simulink library "r2daq_blocks"  (R2012b)
settings: Solver=ode45  StartTime=0.0  StopTime=10.0  RelTol=1e-3
undefined symbols (not defined in the file or in its folder): biquad_iir, feedback_iir, filters, libddc, sfp, synth, xlfir_8x16
libraries: xbsIndex_r4 x4087, casper_library_misc x21, dspsigops x16, casper_library_delays x10, xps_library x1
(part 1 of 23)
settings Model: Creator=ayoung  LastModifiedBy=brent

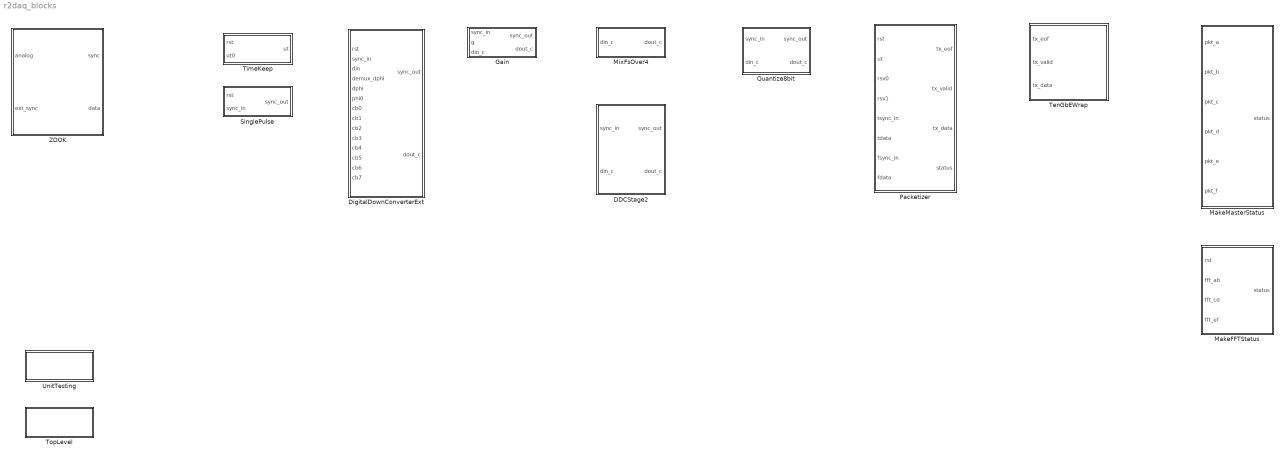
== system r2daq_blocks ==
  DDCStage2 : Subsystem
  DigitalDownConverterExt : Subsystem
  Gain : Subsystem
  MakeFFTStatus : Subsystem
  MakeMasterStatus : Subsystem
  MixFsOver4 : Subsystem
  Packetizer : Subsystem  mask(Packetizer){N_fft=8192, frames_per_batch=390625, IF_ID=1, Digital_ID=3, pd_in=3, pd_tvf=32}
      mask prompts: N_fft "FFT-size"; frames_per_batch "Frames in batch"; IF_ID "IF ID (6-bit)"; Digital_ID "Digital ID (6-bit)"; pd_in "Pipeline delay registers"; pd_tvf "Time packet delay relative to frequency packet"
      mask help:
      | Packetizes simultaneous time- and frequency-domain data for transmission using a 10GbE core.
      |
      | An asynchronous reset port is available as rst.
      |
      | Complex-valued frequency-domain data is supplied as UFix_16_0 to fdata. A single pulse on fsync_in indicates that the first sample of valid data will appear at fdata on the next clock cycle. Only one such pulse should be given per reset. The same applies to tdata and tsync_in.
      |
      | Current unix-time can be supplied as a UFix_32_0 to port ut.
      |
      | 64bit-wide header data can be supplied to each rsv0 and rsv1. Note that b63 (msb) of rsv1 is over-written internally.
      |
      | Signals to drive a 10GbE core are directly available in tx_eof, tx_valid, and tx_data.
      |
      | Empty and full signals of internal FIFO's used to buffer time- and frequency-domain data are available in ffifo_empty, ffifo_full, tfifo_empty and tfifo_full.
      mask init:
      | pd_inst = {...
      |     [gcb '/pd_ud0'],...
      |     [gcb '/pd_ud1']};
      | pd_in = get_param(gcb,'pd_in');
      | for ii=1:numel(pd_inst)
      |     set_param(pd_inst{ii},'latency',pd_in);
      | end
      | pd_inst = [gcb '/pd_dtf'];
      | %pd_tvf = get_param(gcb,'pd_tvf');
      | %set_param(pd_inst,'latency',pd_tvf);
      | pd_tvf_delay = 4;
      | set_param([gcb '/data_per_frame'],'const',num2str(N_fft-1));
      | set_param([gcb '/fpb_const'],'const',num2str(frames_per_batch));
      | set_param([gcb '/pd_dtf_pre'],'latency',num2str(pd_tvf_delay));
      | set_param([gcb '/delay_neg_edge'],'latency',num2str(pd_tvf-2*pd_tvf_delay));
      | set_param([gcb '/pd_dtf_post'],'latency',num2str(pd_tvf_delay));
  Quantize8bit : Subsystem  mask(Quantize8bit){pd_io=0}
      mask prompts: pd_io "Pipeline delay"
      mask help:
      | Quantize complex-valued input to Fix_8_7 by slicing top 8bits from each component.
      |
      | Pipeline delay is configurable.
      mask init:
      | pd_inst = {...
      |     [gcb '/pd_sync'],...
      |     [gcb '/pd_data']};
      | pd_io = get_param(gcb,'pd_io');
      | for ii=1:numel(pd_inst)
      |     set_param(pd_inst{ii},'latency',pd_io);
      | end
  SinglePulse : Subsystem
  TenGbEWrap : Subsystem  mask(TenGbEWrap){pd_in=3, pd_out=3}
      mask prompts: pd_in "Registers in pipeline delay"; pd_out "Registers out pipeline delay"
      mask help:
      | Wrap 10GbE core and supplies control and status registers internally.
      |
      | Pipeline delay to and from registers are configurable.
      mask init:
      | pd_inst = {...
      |     [gcb '/pd_ctrl'],...
      |     [gcb '/pd_port'],...
      |     [gcb '/pd_ip']};
      | pd_in = get_param(gcb,'pd_in');
      | for ii=1:numel(pd_inst)
      |     set_param(pd_inst{ii},'latency',pd_in);
      | end
      | pd_inst = {...
      |     [gcb '/pd_status']};
      | pd_out = get_param(gcb,'pd_out');
      | for ii=1:numel(pd_inst)
      |     set_param(pd_inst{ii},'latency',pd_out);
      | end
  TimeKeep : Subsystem
  TopLevel : Subsystem
      settings: OpenFcn=top_level
  UnitTesting : Subsystem
      settings: OpenFcn=unit_testing
  ZDOK : Subsystem  mask{zdok_slot=ZDOK 1, freq_nyq=1600}
      mask prompts: zdok_slot "ZDOK slot"; freq_nyq "Nyquist frequency [MHz]"
      mask init:
      | adc_inst = [gcb '/asiaa_adc5g'];
      | set_param(adc_inst,'adc_brd',get_param(gcb,'zdok_slot'));
      | set_param(adc_inst,'adc_clk_rate',get_param(gcb,'freq_nyq'));
      mask TypeOptions zdok_slot: ZDOK 0 | ZDOK 1

== system r2daq_blocks/DDCStage2 ==
  sync_in : Inport
  din_c : Inport  Port=2
  biquad_iir1 : Subsystem  AncestorBlock=filters/biquad_iir  mask(biquad_iir){n_bits_in=25, bin_pt_in=16, n_bits_coeff=18, bin_pt_coeff=16, n_bits_out=25, bin_pt_out=16, b_vec=|, a_vec=|}
      mask b_vec=|
      | [0.815263251415296
      |    0.303032070623539
      |    0.115081529740996
      |   -0.260678104245120
      |   -1.000000000000000
      |   -0.139222121675215
      |   -0.134747469852716
      |    0.133883526675981
      |    0.409233506038348]
      mask a_vec=|
      | [1.000000000000000
      |                    0
      |                    0
      |                    0
      |   -1.169556335764851
      |                    0
      |                    0
      |                    0
      |    0.398930973732319]
      mask prompts: n_bits_in "Input bit width"; bin_pt_in "Input decimal point"; n_bits_coeff "Coefficients bit width"; bin_pt_coeff "Coefficients decimal point"; n_bits_out "Output bit width"; bin_pt_out "Output decimal point"; b_vec "B-coefficients"; a_vec "A-coefficients"
      mask help:
      | Implement an IIR-filter biquad-structure,
      |     dout_c(n) = b0*din_c(n) + b1*din_c(n-1) + b2*din_c(n-2)
      |                   - aN*dout_c(n-N) - a2N*dout_c(n-2*N),
      | where B- and A-coefficients are all real and the input is complex.
      |
      | The implementation assumes a biquad-structure rearranged using scattered-lookahead so that the minimum feedback delay is an integer multiple of N. The B-coefficient vector can be of arbitrary length, while the A-coefficient vector has to be of the form
      |     a_vec = [1.0 zeros(1,N) aN zeros(1,N) a2N].
      |
      | See mask documenation for feedback_iir for more details.
      mask init:
      | biquad_iir_init(gcb, ...
      |     'n_bits_in', n_bits_in, ...
      |     'bin_pt_in', bin_pt_in, ...
      |     'n_bits_coeff', n_bits_coeff, ...
      |     'bin_pt_coeff', bin_pt_coeff, ...
      |     'n_bits_out', n_bits_out, ...
      |     'bin_pt_out', bin_pt_out, ...
      |     'b_vec', b_vec, ...
      |     'a_vec', a_vec);
  biquad_iir2 : Subsystem  AncestorBlock=filters/biquad_iir  mask(biquad_iir){n_bits_in=25, bin_pt_in=16, n_bits_coeff=18, bin_pt_coeff=16, n_bits_out=25, bin_pt_out=16, b_vec=|, a_vec=|}
      mask b_vec=|
      | [0.675286360138315
      |    1.000000000000000
      |    0.516957329321165
      |   -0.197096849522316
      |   -0.125512805310079
      |   -0.023487042819110
      |   -0.018488842780882
      |    0.004875263881930
      |    0.003748246302952]
      mask a_vec=|
      | [1.000000000000000
      |                    0
      |                    0
      |                    0
      |   -0.061636440918663
      |                    0
      |                    0
      |                    0
      |    0.000982773697858]
      mask prompts: n_bits_in "Input bit width"; bin_pt_in "Input decimal point"; n_bits_coeff "Coefficients bit width"; bin_pt_coeff "Coefficients decimal point"; n_bits_out "Output bit width"; bin_pt_out "Output decimal point"; b_vec "B-coefficients"; a_vec "A-coefficients"
      mask help:
      | Implement an IIR-filter biquad-structure,
      |     dout_c(n) = b0*din_c(n) + b1*din_c(n-1) + b2*din_c(n-2)
      |                   - aN*dout_c(n-N) - a2N*dout_c(n-2*N),
      | where B- and A-coefficients are all real and the input is complex.
      |
      | The implementation assumes a biquad-structure rearranged using scattered-lookahead so that the minimum feedback delay is an integer multiple of N. The B-coefficient vector can be of arbitrary length, while the A-coefficient vector has to be of the form
      |     a_vec = [1.0 zeros(1,N) aN zeros(1,N) a2N].
      |
      | See mask documenation for feedback_iir for more details.
      mask init: same as r2daq_blocks/DDCStage2/biquad_iir1
  mix_fs_over_4 : Subsystem
  sync_out : Outport
  dout_c : Outport  Port=2
  wires:
  din_c/1 -> mix_fs_over_4/1(din_c)
  sync_in/1 -> biquad_iir1/1(sync_in)
  mix_fs_over_4/1(dout_c) -> biquad_iir1/2(din_c)
  biquad_iir1/1(sync_out) -> biquad_iir2/1(sync_in)
  biquad_iir1/2(dout_c) -> biquad_iir2/2(din_c)
  biquad_iir2/1(sync_out) -> sync_out/1
  biquad_iir2/2(dout_c) -> dout_c/1

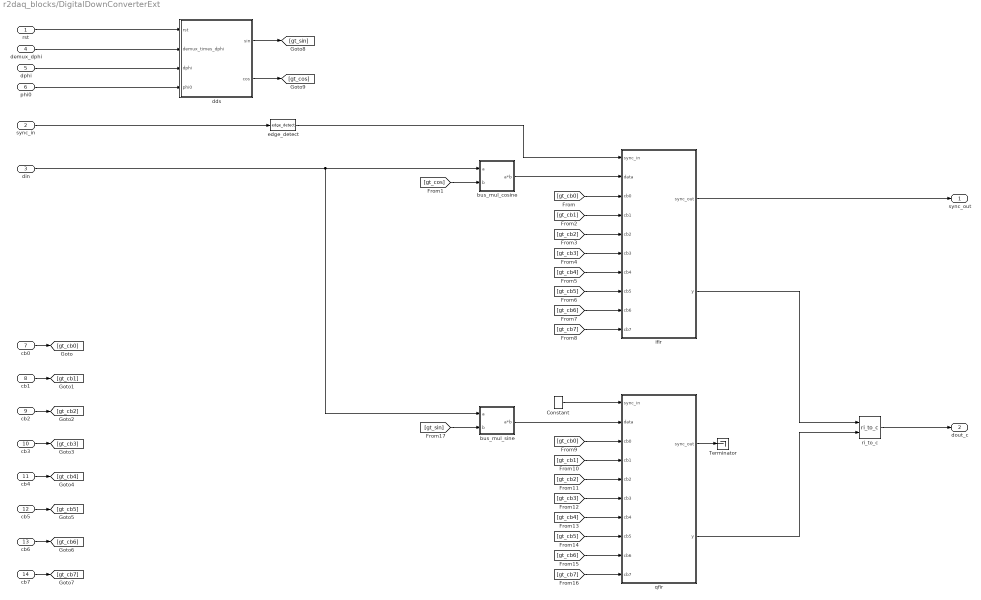
== system r2daq_blocks/DigitalDownConverterExt ==
  rst : Inport
  sync_in : Inport  Port=2
  din : Inport  Port=3
  demux_dphi : Inport  Port=4
  dphi : Inport  Port=5
  phi0 : Inport  Port=6
  cb0 : Inport  Port=7
  cb1 : Inport  Port=8
  cb2 : Inport  Port=9
  cb3 : Inport  Port=10
  cb4 : Inport  Port=11
  cb5 : Inport  Port=12
  cb6 : Inport  Port=13
  cb7 : Inport  Port=14
  Constant : xbsIndex_r4/Constant  const=0  gui_display_data_type=Boolean  arith_type=Boolean  n_bits=16  bin_pt=14  preci_type=Single  exp_width=8  frac_width=24  explicit_period=on  period=1  equ=P=C  opselect=C  inp2=PCIN>>17  opr=+  inp1=P  carry=CIN  dbl_ovrd=off  block_type=constant
  Terminator : Terminator
  bus_mul_cosine : Subsystem  AncestorBlock=casper_library_bus/bus_mult  mask(bus_mult){n_bits_a=ones(1,16)*8, bin_pt_a=ones(1,16)*7, type_a=ones(1,16)*1, cmplx_a=off, n_bits_b=ones(1,16)*11, bin_pt_b=ones(1,16)*9, type_b=ones(1,16)*1, cmplx_b=off, n_bits_out=ones(1,16)*18, bin_pt_out=ones(1,16)*16, type_out=ones(1,16)*1, quantization=0, overflow=0, mult_latency=3, add_latency=1, conv_latency=1, max_fanout=2, fan_latency=0, multiplier_implementation=behavioral HDL, misc=off}
      mask prompts: n_bits_a "a input bit widths"; bin_pt_a "a input binary points"; type_a "a input type (Unsigned=0, Signed=1)"; cmplx_a "a input complex"; n_bits_b "b input bit widths"; bin_pt_b "b input binary points"; type_b "b input type (Unsigned=0, Signed=1)"; cmplx_b "b input complex"; n_bits_out "output bit widths"; bin_pt_out "output binary points"; type_out "output type (Unsigned=0, Signed=1)"; quantization "quantization strategy (Truncate=0, Round  (unbiased: +/- Inf)=1)"; overflow "overflow strategy (Wrap=0, Saturate=1, Flag as error=2)"; mult_latency "multiplier latency"; add_latency "adder latency"; conv_latency "convert latency"; max_fanout "limit fanout to ?"; fan_latency "fanout register latency"; multiplier_implementation "multiplier implementation"; misc "misc support"
      mask help: Multiply components of two busses
      mask init:
      | bus_mult_init(gcb, ...
      |     'n_bits_a', n_bits_a, ...
      |     'bin_pt_a', bin_pt_a, ...
      |     'type_a', type_a, ...
      |     'cmplx_a', cmplx_a, ...
      |     'n_bits_b', n_bits_b, ...
      |     'bin_pt_b', bin_pt_b, ...
      |     'type_b', type_b, ...
      |     'cmplx_b', cmplx_b, ...
      |     'n_bits_out', n_bits_out, ...
      |     'bin_pt_out', bin_pt_out, ...
      |     'type_out', type_out, ...
      |     'quantization', quantization, ...
      |     'overflow', overflow, ...
      |     'mult_latency', mult_latency, ...
      |     'add_latency', add_latency, ...
      |     'conv_latency', conv_latency, ...
      |     'max_fanout', max_fanout, ...
      |     'fan_latency', fan_latency, ...
      |     'multiplier_implementation', multiplier_implementation, ...
      |     'misc', misc);
      mask TypeOptions multiplier_implementation: behavioral HDL | standard core | embedded multiplier core
  bus_mul_sine : Subsystem  AncestorBlock=casper_library_bus/bus_mult  mask(bus_mult){n_bits_a=ones(1,16)*8, bin_pt_a=ones(1,16)*7, type_a=ones(1,16)*1, cmplx_a=off, n_bits_b=ones(1,16)*11, bin_pt_b=ones(1,16)*9, type_b=ones(1,16)*1, cmplx_b=off, n_bits_out=ones(1,16)*18, bin_pt_out=ones(1,16)*16, type_out=ones(1,16)*1, quantization=0, overflow=0, mult_latency=3, add_latency=1, conv_latency=1, max_fanout=2, fan_latency=0, multiplier_implementation=behavioral HDL, misc=off}
      mask prompts: n_bits_a "a input bit widths"; bin_pt_a "a input binary points"; type_a "a input type (Unsigned=0, Signed=1)"; cmplx_a "a input complex"; n_bits_b "b input bit widths"; bin_pt_b "b input binary points"; type_b "b input type (Unsigned=0, Signed=1)"; cmplx_b "b input complex"; n_bits_out "output bit widths"; bin_pt_out "output binary points"; type_out "output type (Unsigned=0, Signed=1)"; quantization "quantization strategy (Truncate=0, Round  (unbiased: +/- Inf)=1)"; overflow "overflow strategy (Wrap=0, Saturate=1, Flag as error=2)"; mult_latency "multiplier latency"; add_latency "adder latency"; conv_latency "convert latency"; max_fanout "limit fanout to ?"; fan_latency "fanout register latency"; multiplier_implementation "multiplier implementation"; misc "misc support"
      mask help: Multiply components of two busses
      mask init: same as r2daq_blocks/DigitalDownConverterExt/bus_mul_cosine
      mask TypeOptions multiplier_implementation: behavioral HDL | standard core | embedded multiplier core
  dds : Subsystem  AncestorBlock=libddc/synth  mask(synth){n_parout=16, sum_latency=1, n_ph_bits=10, n_amp_bits=11, out_type=Sine and Cosine}
      mask prompts: n_parout "Number of parallel outputs"; sum_latency "Latency (sum)"; n_ph_bits "Bitwidth phase"; n_amp_bits "Bitwidth amplitude"; out_type "Requested outputs"
      mask help:
      | Implements a DDS with demuxed output and reconfigurable phase and frequency.
      |
      | Number of parallel outputs should be at least 2.
      |
      | Adder latencies can be specified, and the overall latency of the DDS is displayed.
      mask init:
      | synth_init(gcb,...
      | 'n_parout',n_parout,...
      | 'sum_latency',sum_latency,...
      | 'n_ph_bits',n_ph_bits,...
      | 'n_amp_bits',n_amp_bits,...
      | 'out_type',out_type ...
      | );
      mask Help: Nothing here yet.
      mask TypeOptions out_type: Sine and Cosine | Sine | Cosine
  edge_detect : casper_library_misc/edge_detect  edge=Rising  polarity=Active High  x_in=[0 0.08 0.08 0.16 0.16 0.24 0.24 0.32 0.32 0.4]  y_in="[-1 -1  1  1  1  1  1  1  1  1]"  x_out=[0.6 0.68 0.68 0.76 0.76 0.84 0.84 0.92 0.92 1]  y_out="[-1 -1  1  1 -1 -1 -1 -1 -1 -1]"
  ifir : Subsystem  AncestorBlock=libddc/xlfir_8x16  mask(xlfir_8x16){n_bits_data=18, bin_pt_data=16, n_bits_coeff=8, bin_pt_coeff=7, n_bits_out=25, bin_pt_out=16}
      mask prompts: n_bits_data "Data bit widths"; bin_pt_data "Data binary points"; n_bits_coeff "Coefficient bit widths"; bin_pt_coeff "Coefficient binary points"; n_bits_out "Output bit widths (adder tree bit-growth is 7)"; bin_pt_out "Output binary ponits"
      mask help:
      | Implement a 127-order FIR with 16x demuxed input (128 coefficients)
      |
      |     y = b0*x[n] + b1*x[n-1] + b2*x[n-2] + ... + b127*x[n-127].
      |
      | Data is presented on a single bus. Coefficients are presented in groups of 16 on each of 8 busses.
      |
      | The coefficients are presented as follows
      |
      |     cb0[msb ... lsb] = [b15 ... b0]
      |     cb1[msb ... lsb] = [b31 ... b16]
      |     ...
      |
      | and so on.
      mask init:
      | xlfir_8x16_init(gcb, ...
      |     'n_bits_data', n_bits_data, ...
      |     'bin_pt_data', bin_pt_data, ...
      |     'n_bits_coeff', n_bits_coeff, ...
      |     'bin_pt_coeff', bin_pt_coeff, ...
      |     'n_bits_out', n_bits_out, ...
      |     'bin_pt_out', bin_pt_out);
  qfir : Subsystem  AncestorBlock=libddc/xlfir_8x16  mask(xlfir_8x16){n_bits_data=18, bin_pt_data=16, n_bits_coeff=8, bin_pt_coeff=7, n_bits_out=25, bin_pt_out=16}
      mask prompts: n_bits_data "Data bit widths"; bin_pt_data "Data binary points"; n_bits_coeff "Coefficient bit widths"; bin_pt_coeff "Coefficient binary points"; n_bits_out "Output bit widths (adder tree bit-growth is 7)"; bin_pt_out "Output binary ponits"
      mask help:
      | Implement a 127-order FIR with 16x demuxed input (128 coefficients)
      |
      |     y = b0*x[n] + b1*x[n-1] + b2*x[n-2] + ... + b127*x[n-127].
      |
      | Data is presented on a single bus. Coefficients are presented in groups of 16 on each of 8 busses.
      |
      | The coefficients are presented as follows
      |
      |     cb0[msb ... lsb] = [b15 ... b0]
      |     cb1[msb ... lsb] = [b31 ... b16]
      |     ...
      |
      | and so on.
      mask init: same as r2daq_blocks/DigitalDownConverterExt/ifir
  ri_to_c : casper_library_misc/ri_to_c
  sync_out : Outport
  dout_c : Outport  Port=2
  wires:
  cb0/1 -> [gt_cb0]
  cb1/1 -> [gt_cb1]
  cb2/1 -> [gt_cb2]
  cb3/1 -> [gt_cb3]
  cb4/1 -> [gt_cb4]
  cb5/1 -> [gt_cb5]
  cb6/1 -> [gt_cb6]
  cb7/1 -> [gt_cb7]
  dds/2(cos) -> [gt_cos]
  dds/1(sin) -> [gt_sin]
  [gt_cb0] -> ifir/3(cb0)
  [gt_cb1] -> ifir/4(cb1)
  [gt_cb3] -> ifir/6(cb3)
  [gt_cb4] -> ifir/7(cb4)
  [gt_cb5] -> ifir/8(cb5)
  [gt_cb6] -> ifir/9(cb6)
  bus_mul_cosine/1(a*b) -> ifir/2(data)
  [gt_cb2] -> ifir/5(cb2)
  [gt_cb7] -> ifir/10(cb7)
  edge_detect/1 -> ifir/1(sync_in)
  [gt_cos] -> bus_mul_cosine/2(b)
  [gt_cb0] -> qfir/3(cb0)
  [gt_cb1] -> qfir/4(cb1)
  [gt_cb3] -> qfir/6(cb3)
  [gt_cb4] -> qfir/7(cb4)
  [gt_cb5] -> qfir/8(cb5)
  [gt_cb6] -> qfir/9(cb6)
  [gt_cb2] -> qfir/5(cb2)
  [gt_cb7] -> qfir/10(cb7)
  bus_mul_sine/1(a*b) -> qfir/2(data)
  din/1 -> bus_mul_sine/1(a), bus_mul_cosine/1(a)
  [gt_sin] -> bus_mul_sine/2(b)
  rst/1 -> dds/1(rst)
  sync_in/1 -> edge_detect/1
  ifir/1(sync_out) -> sync_out/1
  qfir/2(y) -> ri_to_c/2
  qfir/1(sync_out) -> Terminator/1
  Constant/1 -> qfir/1(sync_in)
  demux_dphi/1 -> dds/2(demux_times_dphi)
  dphi/1 -> dds/3(dphi)
  phi0/1 -> dds/4(phi0)
  ifir/2(y) -> ri_to_c/1
  ri_to_c/1 -> dout_c/1

== system r2daq_blocks/Gain ==
  sync_in : Inport
  g : Inport  Port=2
  din_c : Inport  Port=3
  Delay : xbsIndex_r4/Delay  rst=off  infoeditControl=Selection of Reset will increase slice count due to use of real FFs and instead of SRLs  en=off  latency=3  dbl_ovrd=off  reg_retiming=off  block_type=delay
  c_to_ri : casper_library_misc/c_to_ri  n_bits=25  bin_pt=16
      settings: AttributesFormatString=25_16 r/i
  mul_im : xbsIndex_r4/Mult  precision=User Defined  arith_type="Signed  (2's comp)"  n_bits=25  bin_pt=16  quantization="Round  (unbiased: +/- Inf)"  overflow=Saturate  en=off  latency=3  dbl_ovrd=off  use_behavioral_HDL=off  opt=Speed  use_embedded=on  optimum_pipeline=off  pipeline=on  use_rpm=on  placement_style=Triangular  block_type=mult
  mul_re : xbsIndex_r4/Mult  precision=User Defined  arith_type="Signed  (2's comp)"  n_bits=25  bin_pt=16  quantization="Round  (unbiased: +/- Inf)"  overflow=Saturate  en=off  latency=3  dbl_ovrd=off  use_behavioral_HDL=off  opt=Speed  use_embedded=on  optimum_pipeline=off  pipeline=on  use_rpm=on  placement_style=Triangular  block_type=mult
  ri_to_c : casper_library_misc/ri_to_c
  sync_out : Outport
  dout_c : Outport  Port=2
  wires:
  g/1 -> mul_im/1, mul_re/1
  c_to_ri/1 -> mul_re/2
  c_to_ri/2 -> mul_im/2
  din_c/1 -> c_to_ri/1
  mul_re/1 -> ri_to_c/1
  mul_im/1 -> ri_to_c/2
  ri_to_c/1 -> dout_c/1
  sync_in/1 -> Delay/1
  Delay/1 -> sync_out/1

== system r2daq_blocks/MakeFFTStatus ==
  rst : Inport
  fft_ab : Inport  Port=2
  fft_cd : Inport  Port=3
  fft_ef : Inport  Port=4
  Concat : xbsIndex_r4/Concat  num_inputs=4  dbl_ovrd=off  block_type=concat
  cnt_ab : xbsIndex_r4/Counter  cnt_type=Free Running  cnt_to=Inf  operation=Up  start_count=0  cnt_by_val=1  arith_type=Unsigned  n_bits=10  bin_pt=0  load_pin=off  rst=on  en=on  explicit_period=on  period=1  dbl_ovrd=off  use_behavioral_HDL=off  implementation=Fabric  block_type=counter
  cnt_cd : xbsIndex_r4/Counter  cnt_type=Free Running  cnt_to=Inf  operation=Up  start_count=0  cnt_by_val=1  arith_type=Unsigned  n_bits=10  bin_pt=0  load_pin=off  rst=on  en=on  explicit_period=on  period=1  dbl_ovrd=off  use_behavioral_HDL=off  implementation=Fabric  block_type=counter
  cnt_cd1 : xbsIndex_r4/Counter  cnt_type=Free Running  cnt_to=Inf  operation=Up  start_count=0  cnt_by_val=1  arith_type=Unsigned  n_bits=10  bin_pt=0  load_pin=off  rst=on  en=on  explicit_period=on  period=1  dbl_ovrd=off  use_behavioral_HDL=off  implementation=Fabric  block_type=counter
  zero : xbsIndex_r4/Constant  const=0  gui_display_data_type=Fixed-point  arith_type=Unsigned  n_bits=2  bin_pt=0  preci_type=Single  exp_width=8  frac_width=24  explicit_period=off  period=1  equ=P=C  opselect=C  inp2=PCIN>>17  opr=+  inp1=P  carry=CIN  dbl_ovrd=off  block_type=constant
  status : Outport
  wires:
  fft_ab/1 -> cnt_ab/2
  fft_cd/1 -> cnt_cd/2
  fft_ef/1 -> cnt_cd1/2
  rst/1 -> cnt_cd/1, cnt_cd1/1, cnt_ab/1
  cnt_cd1/1 -> Concat/4
  cnt_cd/1 -> Concat/3
  cnt_ab/1 -> Concat/2
  zero/1 -> Concat/1
  Concat/1 -> status/1

== system r2daq_blocks/MakeMasterStatus ==
  pkt_a : Inport
  pkt_b : Inport  Port=2
  pkt_c : Inport  Port=3
  pkt_d : Inport  Port=4
  pkt_e : Inport  Port=5
  pkt_f : Inport  Port=6
  Concat : xbsIndex_r4/Concat  num_inputs=6  dbl_ovrd=off  block_type=concat
  status : Outport
  wires:
  pkt_c/1 -> Concat/3
  pkt_d/1 -> Concat/4
  pkt_e/1 -> Concat/5
  pkt_f/1 -> Concat/6
  Concat/1 -> status/1
  pkt_a/1 -> Concat/1
  pkt_b/1 -> Concat/2

== system r2daq_blocks/MixFsOver4 ==
  din_c : Inport
  Counter : xbsIndex_r4/Counter  cnt_type=Free Running  cnt_to=Inf  operation=Up  start_count=0  cnt_by_val=1  arith_type=Unsigned  n_bits=2  bin_pt=0  load_pin=off  rst=off  en=off  explicit_period=on  period=1  dbl_ovrd=off  use_behavioral_HDL=off  implementation=Fabric  block_type=counter
  Negate : xbsIndex_r4/Negate  precision=User Defined  arith_type="Signed  (2's comp)"  n_bits=25  bin_pt=16  quantization="Round  (unbiased: +/- Inf)"  overflow=Saturate  en=off  latency=0  dbl_ovrd=off  block_type=negate
  Negate1 : xbsIndex_r4/Negate  precision=User Defined  arith_type="Signed  (2's comp)"  n_bits=25  bin_pt=16  quantization="Round  (unbiased: +/- Inf)"  overflow=Saturate  en=off  latency=0  dbl_ovrd=off  block_type=negate
  c_to_ri : casper_library_misc/c_to_ri  n_bits=25  bin_pt=16
      settings: AttributesFormatString=25_16 r/i
  im_out : xbsIndex_r4/Mux  inputs=4  en=off  latency=0  precision=User Defined  arith_type=Unsigned  n_bits=25  bin_pt=16  quantization=Truncate  overflow=Wrap  dbl_ovrd=off  block_type=mux
  re_out : xbsIndex_r4/Mux  inputs=4  en=off  latency=0  precision=User Defined  arith_type=Unsigned  n_bits=25  bin_pt=16  quantization=Truncate  overflow=Wrap  dbl_ovrd=off  block_type=mux
  ri_to_c : casper_library_misc/ri_to_c
  dout_c : Outport
  wires:
  din_c/1 -> c_to_ri/1
  ri_to_c/1 -> dout_c/1
  re_out/1 -> ri_to_c/1
  im_out/1 -> ri_to_c/2
  c_to_ri/2 -> [im_p], Negate1/1
  c_to_ri/1 -> [re_p], Negate/1
  Negate/1 -> [re_n]
  Negate1/1 -> [im_n]
  Counter/1 -> [sel]
  [im_p] -> re_out/3
  [re_p] -> re_out/2
  [re_n] -> re_out/4
  [im_n] -> re_out/5
  [sel] -> re_out/1
  [im_n] -> im_out/4
  [im_p] -> im_out/2
  [re_p] -> im_out/5
  [sel] -> im_out/1
  [re_n] -> im_out/3
